simulink model "blood_pressure_measurement"  (R2022b)
settings: Solver=VariableStepAuto  StartTime=0.0  StopTime=10.0  RelTol=1e-3
libraries: arduinolib x3, simulink x1
settings Model: Creator=Menath  LastModifiedBy=Menath

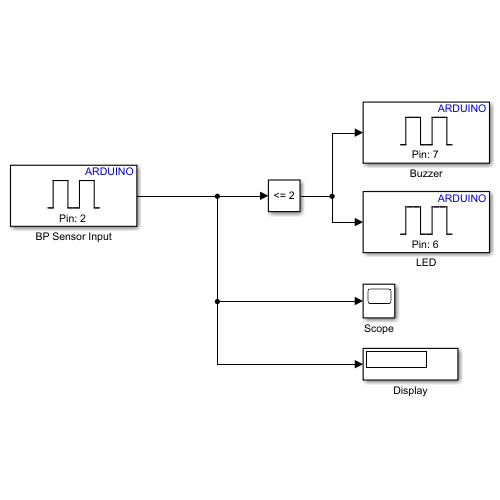
[thumbnail: Simulink's stored preview of the top-level diagram]
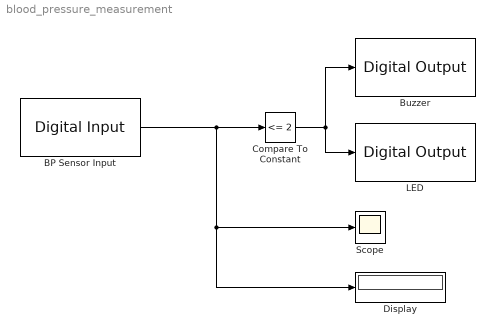
== system blood_pressure_measurement ==
  BP Sensor Input : arduinolib/Digital Input  pinNumber=2  mode=Default  Direction=input  SampleTime=0.1  blockPlatform=arduino
  Buzzer : arduinolib/Digital Output  pinNumber=7  Direction=output  blockPlatform=arduino
  Compare To Constant : simulink/Logic and Bit Operations/Compare To Constant  relop=<=  const=2  OutDataTypeStr=boolean
  Display : Display
  LED : arduinolib/Digital Output  pinNumber=6  Direction=output  blockPlatform=arduino
  Scope : Scope
  wires:
  Compare To Constant/1 -> LED/1, Buzzer/1
  BP Sensor Input/1 -> Display/1, Scope/1, Compare To Constant/1
